simulink subsystem "FeedForward"  (R2024b)
settings: Solver=VariableStepAuto  StartTime=0.0  StopTime=10.0  RelTol=1e-3
model mask{rwheel=0, L=0, StrWhlRatio=0, Izz=0, tr=0, Gr=0, MotorT=0, MotorW=0, Tf=0, Tmax=0, Ku=0}
  mask prompts: rwheel "Wheel Radius"; L "Wheelbase"; StrWhlRatio "Steering Ratio"; Izz "Ineritia Around Z"; tr "Rear Track"; Gr "Gear Ratio"; MotorT "Motor Map Torque"; MotorW "Motor Map RPM"; Tf "Low Pass Filter Time const"; Tmax "Max Torque"; Ku "Understeer Gradient"
values from neighbouring files (symbols this model uses):
  Gr = 1/Vehicle.Powertrain.Driveline.GearboxR2.ratio.Value    [sm_car_controlparam_FeedF.m]
  L = -Vehicle.Chassis.Body.sAxle2.Value(1)    [sm_car_controlparam_FeedF.m]
  rwheel = tire_param.DIMENSION.UNLOADED_RADIUS    [sm_car_controlparam_FeedF.m]
  tr = Vehicle.Chassis.Body.TrackRear.Value    [sm_car_controlparam_FeedF.m]
libraries: simulink x4, simulink_extras x1
settings Model: Creator=andrei  LastModifiedBy=andrei

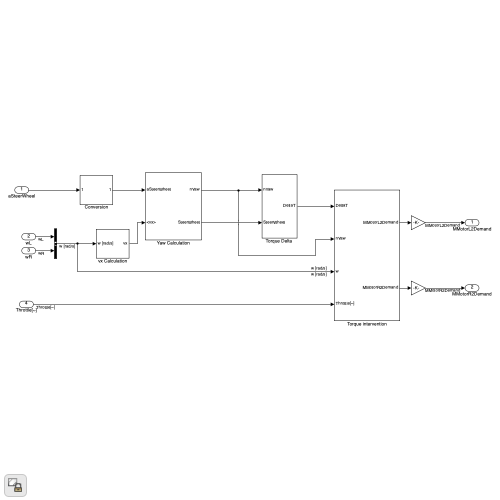
[thumbnail: Simulink's stored preview of the top-level diagram]
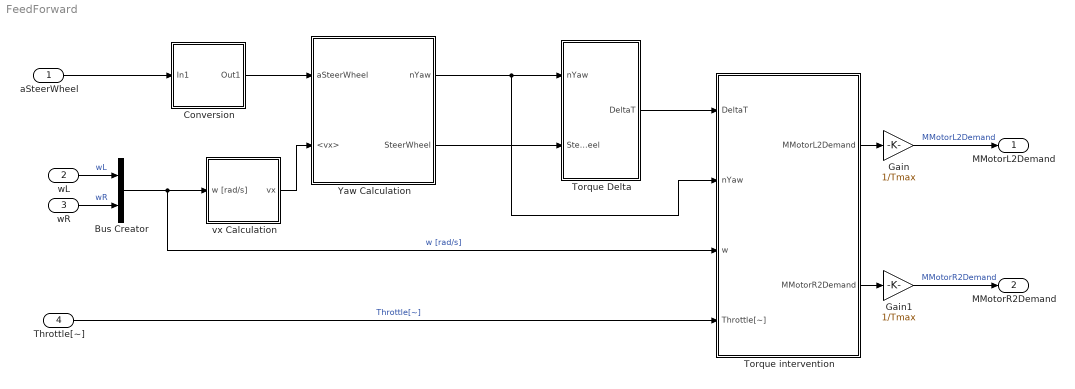
== system FeedForward ==
  aSteerWheel : Inport  OutDataTypeStr=double  PortDimensions=1  SampleTime=0
  wL : Inport  Port=2  OutDataTypeStr=double  PortDimensions=1  SampleTime=0
  wR : Inport  Port=3  OutDataTypeStr=double  PortDimensions=1  SampleTime=0
  Throttle[~] : Inport  Port=4  OutDataTypeStr=double  PortDimensions=1  SampleTime=0
  Bus Creator : BusCreator  Inputs=2
  Conversion : Subsystem
  Gain : Gain  Gain=1/Tmax
  Gain1 : Gain  Gain=1/Tmax
  "Torque Delta " : Subsystem
  Torque intervention : Subsystem
  Yaw Calculation : Subsystem
  vx Calculation : Subsystem
  MMotorL2Demand : Outport  OutDataTypeStr=double  PortDimensions=1  SampleTime=0
  MMotorR2Demand : Outport  Port=2  OutDataTypeStr=double  PortDimensions=1  SampleTime=0
  wires:
  Conversion/1(Out1) -> Yaw Calculation/1(aSteerWheel)
  Gain/1 -> MMotorL2Demand/1  "MMotorL2Demand"
  Yaw Calculation/1(nYaw) -> "Torque Delta "/1(nYaw), Torque intervention/2(nYaw)
  wL/1 -> Bus Creator/1  "wL"
  Throttle[~]/1 -> Torque intervention/4(Throttle[~])  "Throttle[~]"
  aSteerWheel/1 -> Conversion/1(In1)
  wR/1 -> Bus Creator/2  "wR"
  Bus Creator/1 -> Torque intervention/3(w), vx Calculation/1(w [rad/s])  "w [rad/s]"
  vx Calculation/1(vx) -> Yaw Calculation/2(<vx>)
  Gain1/1 -> MMotorR2Demand/1  "MMotorR2Demand"
  Yaw Calculation/2(SteerWheel) -> "Torque Delta "/2(SteerWheel)
  Torque intervention/1(MMotorL2Demand) -> Gain/1
  Torque intervention/2(MMotorR2Demand) -> Gain1/1
  "Torque Delta "/1(DeltaT) -> Torque intervention/1(DeltaT)

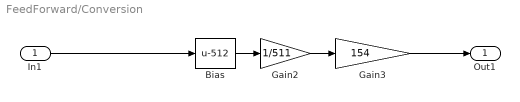
== system FeedForward/Conversion ==
  In1 : Inport
  Bias : Bias  Bias=-512  SaturateOnIntegerOverflow=off
  Gain2 : Gain  Gain=1/511
  Gain3 : Gain  Gain=154
  Out1 : Outport
  wires:
  Gain2/1 -> Gain3/1
  In1/1 -> Bias/1
  Gain3/1 -> Out1/1
  Bias/1 -> Gain2/1

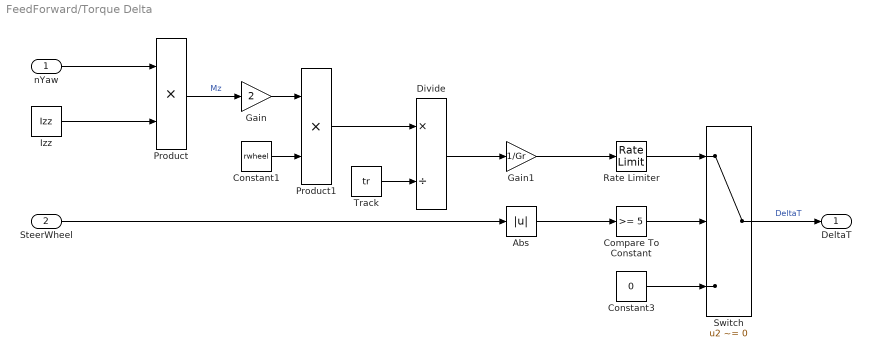
== system FeedForward/Torque Delta  ==
  nYaw : Inport
  SteerWheel : Inport  Port=2
  Abs : Abs  SaturateOnIntegerOverflow=off
  Compare To Constant : simulink/Logic and Bit Operations/Compare To Constant  relop=>=  const=5  OutDataTypeStr=boolean
  Constant1 : Constant  Value=rwheel
  Constant3 : Constant  Value=0
  Divide : Product  Inputs=*/
  Gain : Gain  Gain=2
  Gain1 : Gain  Gain=1/Gr
  Izz : Constant  Value=Izz
  Product : Product
  Product1 : Product
  Rate Limiter : RateLimiter  RisingSlewLimit=60  FallingSlewLimit=-60  SampleTimeMode=inherited
  Switch : Switch  Criteria=u2 ~= 0  SaturateOnIntegerOverflow=off  InputSameDT=off
  "Track " : Constant  Value=tr
  DeltaT : Outport
  wires:
  Abs/1 -> Compare To Constant/1
  Switch/1 -> DeltaT/1  "DeltaT"
  Constant3/1 -> Switch/3
  Compare To Constant/1 -> Switch/2
  SteerWheel/1 -> Abs/1
  Rate Limiter/1 -> Switch/1
  Gain1/1 -> Rate Limiter/1
  Divide/1 -> Gain1/1
  "Track "/1 -> Divide/2
  Product1/1 -> Divide/1
  Constant1/1 -> Product1/2
  Gain/1 -> Product1/1
  Product/1 -> Gain/1  "Mz"
  Izz/1 -> Product/2
  nYaw/1 -> Product/1

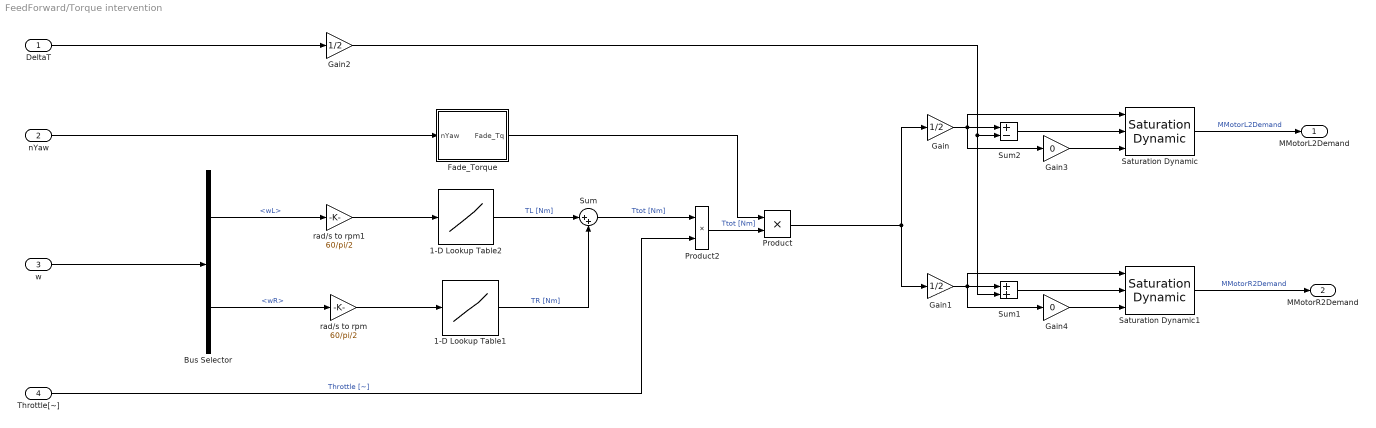
== system FeedForward/Torque intervention ==
  DeltaT : Inport
  nYaw : Inport  Port=2
  w : Inport  Port=3
  Throttle[~] : Inport  Port=4
  1-D Lookup Table1 : Lookup_n-D  NumberOfTableDimensions=1  BreakpointsForDimension1=MotorW  Table=MotorT  InternalRulePriority=Speed  RndMeth=Simplest
  1-D Lookup Table2 : Lookup_n-D  NumberOfTableDimensions=1  BreakpointsForDimension1=MotorW  Table=MotorT  InternalRulePriority=Speed  RndMeth=Simplest
  Bus Selector : BusSelector  OutputSignals=wL,wR
  Fade_Torque : Subsystem
  Gain : Gain  Gain=1/2
  Gain1 : Gain  Gain=1/2
  Gain2 : Gain  Gain=1/2
  Gain3 : Gain  Gain=0
  Gain4 : Gain  Gain=0
  Product : Product
  Product2 : Product
  Saturation Dynamic : simulink/Discontinuities/Saturation Dynamic  OutMin=[]  OutMax=[]  OutDataTypeStr=Inherit: Same as second input  OutDataType=fixdt(1, 16)  OutScaling=2^-10  DoSatur=off
  Saturation Dynamic1 : simulink/Discontinuities/Saturation Dynamic  OutMin=[]  OutMax=[]  OutDataTypeStr=Inherit: Same as second input  OutDataType=fixdt(1, 16)  OutScaling=2^-10  DoSatur=off
  Sum : Sum  Inputs=|++
  Sum1 : Sum
  Sum2 : Sum  Inputs=+-
  rad/s to rpm : Gain  Gain=60/pi/2
  rad/s to rpm1 : Gain  Gain=60/pi/2
  MMotorL2Demand : Outport
  MMotorR2Demand : Outport  Port=2
  wires:
  Product/1 -> Gain1/1, Gain/1
  Fade_Torque/1(Fade_Tq) -> Product/1
  Product2/1 -> Product/2  "Ttot [Nm]"
  nYaw/1 -> Fade_Torque/1(nYaw)
  Gain2/1 -> Sum2/2, Sum1/2
  Gain4/1 -> Saturation Dynamic1/3
  Sum1/1 -> Saturation Dynamic1/2
  Sum2/1 -> Saturation Dynamic/2
  Gain3/1 -> Saturation Dynamic/3
  Saturation Dynamic/1 -> MMotorL2Demand/1  "MMotorL2Demand"
  Saturation Dynamic1/1 -> MMotorR2Demand/1  "MMotorR2Demand"
  Gain1/1 -> Sum1/1, Saturation Dynamic1/1, Gain4/1
  DeltaT/1 -> Gain2/1
  Gain/1 -> Sum2/1, Saturation Dynamic/1, Gain3/1
  Throttle[~]/1 -> Product2/2  "Throttle [~]"
  Sum/1 -> Product2/1  "Ttot [Nm]"
  rad/s to rpm/1 -> 1-D Lookup Table1/1
  rad/s to rpm1/1 -> 1-D Lookup Table2/1
  w/1 -> Bus Selector/1
  Bus Selector/1 -> rad/s to rpm1/1  "<wL>"
  Bus Selector/2 -> rad/s to rpm/1  "<wR>"
  1-D Lookup Table2/1 -> Sum/1  "TL [Nm]"
  1-D Lookup Table1/1 -> Sum/2  "TR [Nm]"

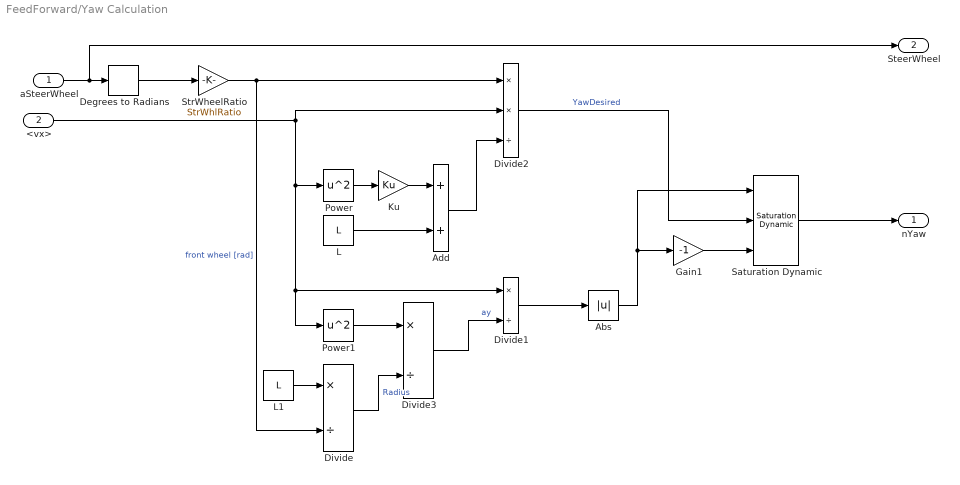
== system FeedForward/Yaw Calculation ==
  aSteerWheel : Inport
  <vx> : Inport  Port=2
  Abs : Abs  SaturateOnIntegerOverflow=off
  Add : Sum
  Degrees to Radians : simulink_extras/Transformations/Degrees to Radians
  Divide : Product  Inputs=*/
  Divide1 : Product  Inputs=*/
  Divide2 : Product  Inputs=**/
  Divide3 : Product  Inputs=*/
  Gain1 : Gain  Gain=-1
  Ku : Gain  Gain=Ku
  L : Constant  Value=L
  L1 : Constant  Value=L
  Power : Math  Operator=square
  Power1 : Math  Operator=square
  Saturation Dynamic : simulink/Discontinuities/Saturation Dynamic  OutMin=[]  OutMax=[]  OutDataTypeStr=Inherit: Same as second input  OutDataType=fixdt(1, 16)  OutScaling=2^-10  DoSatur=off
  StrWheelRatio : Gain  Gain=StrWhlRatio
  nYaw : Outport
  SteerWheel : Outport  Port=2
  wires:
  Degrees to Radians/1 -> StrWheelRatio/1
  Divide/1 -> Divide3/2  "Radius"
  Power1/1 -> Divide3/1
  L1/1 -> Divide/1
  Saturation Dynamic/1 -> nYaw/1
  StrWheelRatio/1 -> Divide2/1, Divide/2  "front wheel [rad]"
  Power/1 -> Ku/1
  Divide2/1 -> Saturation Dynamic/2  "YawDesired"
  Abs/1 -> Saturation Dynamic/1, Gain1/1
  L/1 -> Add/2
  Gain1/1 -> Saturation Dynamic/3
  Ku/1 -> Add/1
  Divide3/1 -> Divide1/2  "ay"
  Divide1/1 -> Abs/1
  <vx>/1 -> Divide2/2, Power/1, Divide1/1, Power1/1
  Add/1 -> Divide2/3
  aSteerWheel/1 -> Degrees to Radians/1, SteerWheel/1

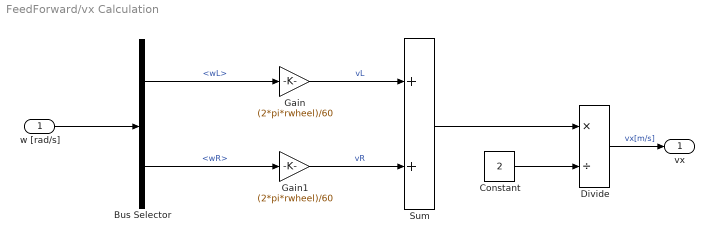
== system FeedForward/vx Calculation ==
  w [rad/s] : Inport
  Bus Selector : BusSelector  OutputSignals=wL,wR
  Constant : Constant  Value=2
  Divide : Product  Inputs=*/
  Gain : Gain  Gain=(2*pi*rwheel)/60
  Gain1 : Gain  Gain=(2*pi*rwheel)/60
  Sum : Sum
  vx : Outport
  wires:
  Constant/1 -> Divide/2
  Divide/1 -> vx/1  "vx[m/s]"
  Sum/1 -> Divide/1
  Gain1/1 -> Sum/2  "vR"
  Gain/1 -> Sum/1  "vL"
  Bus Selector/2 -> Gain1/1  "<wR>"
  Bus Selector/1 -> Gain/1  "<wL>"
  w [rad/s]/1 -> Bus Selector/1

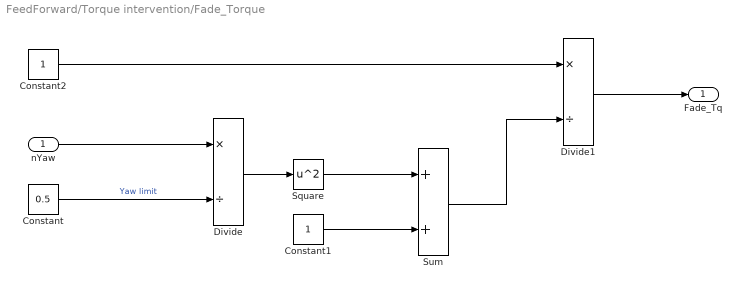
== system FeedForward/Torque intervention/Fade_Torque ==
  nYaw : Inport
  Constant : Constant  Value=0.5
  Constant1 : Constant
  Constant2 : Constant
  Divide : Product  Inputs=*/
  Divide1 : Product  Inputs=*/
  Square : Math  Operator=square
  Sum : Sum
  Fade_Tq : Outport
  wires:
  Divide1/1 -> Fade_Tq/1
  Sum/1 -> Divide1/2
  Constant2/1 -> Divide1/1
  Constant1/1 -> Sum/2
  Square/1 -> Sum/1
  Divide/1 -> Square/1
  Constant/1 -> Divide/2  "Yaw limit"
  nYaw/1 -> Divide/1
